simulink model "gm_uz_pmsm_model_nonlinear"  (R2023a)
settings: Solver=FixedStepAuto  StartTime=0.0  StopTime=0.5  RelTol=1e-3
PreLoadFcn:
  | uz_pmsm_model_init_parameter
PostLoadFcn:
  | % Import the data from Excel for a lookup table
  | FluxMapData = readtable('C:\Users\Philipp\ultrazohm\ultrazohm_sw\ip_cores\uz_pmsm_model\FluxMapData_2023-05-26_13-07-57.csv');
  | % Row indices for lookup table
  | d_current_in_d_axis = FluxMapData(8:27,1:end);
  | % Column indices for lookup table
  | q_current_in_d_axis = FluxMapData(29:48,1:end);
  | % Output values for lookup table
  | d_Flux_d_axis = FluxMapData(50:69,1:end);
undefined symbols (not defined in the file or in its folder): d_current_d_Flux, d_current_q_Flux, Flux_d, Flux_q, friction_coefficient, inertia, k_i_d, k_p_d, k_p_q, L_d, L_q, Ldd, Ldq, Lqd, Lqq, polepair, psi_pm, q_current_d_Flux, q_current_q_Flux, R_1, setpoint_step, simulate_mechanical, simulate_open_loop, static_friction_torque
libraries: hdlmdlgenlib x8, slpidlib x2
(part 1 of 2)
settings Model: Creator=ts  LastModifiedBy=Philipp
settings SolverCC: AlgebraicLoopSolver=TrustRegion  AutoInsertRateTranBlk=on
settings DataIOCC: LimitDataPoints=on  SaveOutput=off  SaveTime=off
settings OptimizationCC: BlockReduction=off  ConditionallyExecuteInputs=off  DefaultParameterBehavior=Inlined  LifeSpan=inf
settings DebuggingCC: AlgebraicLoopMsg=error  InheritedTsInSrcMsg=none  SingleTaskRateTransMsg=error  UnconnectedInputMsg=warning  UnconnectedOutputMsg=warning  UnconnectedLineMsg=warning  AllowSymbolicDim=off  StrictBusMsg=ErrorOnBusTreatedAsVector  SFUnexpectedBacktrackingDiag=warning  SFNoUnconditionalDefaultTransitionDiag=warning  SFExecutionAtInitializationDiag=none  ArithmeticOperatorsInVariantConditions=warning
settings HardwareCC: ProdBitPerPointer=32  ProdBitPerSizeT=32  ProdBitPerPtrDiffT=32  ProdLargestAtomicFloat=None  ProdIntDivRoundTo=Undefined  ProdEndianess=Unspecified  ProdWordSize=32  ProdHWDeviceType=ASIC/FPGA->ASIC/FPGA  ProdEqTarget=off
settings ModelReferenceCC: EnableRefExpFcnMdlSchedulingChecks=on
settings SFSimCC: SimUseLocalCustomCode=off  CustomCodeUndefinedFunction=UseInterfaceOnly
settings RTWCC: RTWUseLocalCustomCode=off  DLArmComputeVersion=19.05
settings CodeAppCC: StateflowObjectComments=on
settings GRTTargetCC: TargetLangStandard=C89/C90 (ANSI)
settings ConfigComp: CovScope=ReferencedModels  CovMetricSettings=dw  CovSaveCumulativeToWorkspaceVar=on  CovSaveSingleToWorkspaceVar=on  CovExternalEMLEnable=off  CovSFcnEnable=off

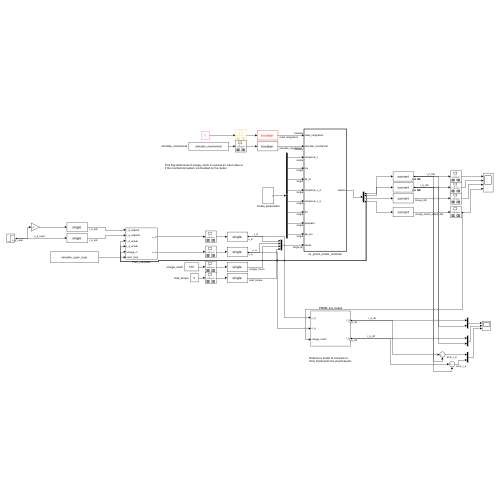
[thumbnail: Simulink's stored preview of the top-level diagram]
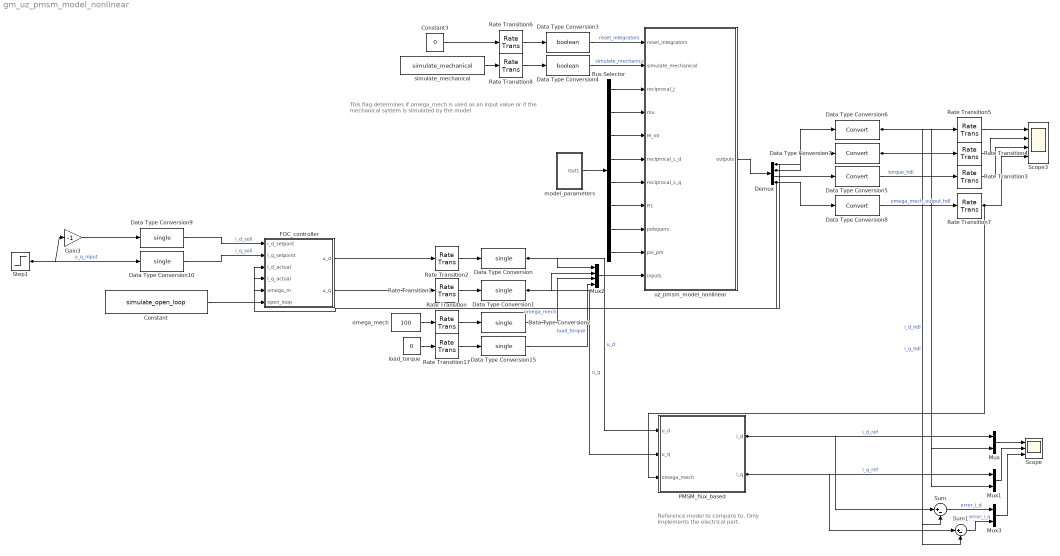
== system gm_uz_pmsm_model_nonlinear ==
  note: This flag determines if omega_mech is used as an input value or
      | if the mechanical system is simulated by the model
  note: Reference model to compare to.
      | Only implements the electrical part.
  Bus Selector : BusSelector  OutputSignals=1_J,mu,M_R0,1_L_d,1_L_q,R_1,polepair,psi_pm
  Constant : Constant  Value=simulate_open_loop
  Constant3 : Constant  Value=0
  Data Type Conversion{,1..2,9..10,15} (6 alike) : DataTypeConversion  OutDataTypeStr=single  SaturateOnIntegerOverflow=off  RndMeth=Floor
  Data Type Conversion3 : DataTypeConversion  OutDataTypeStr=boolean  SaturateOnIntegerOverflow=off  RndMeth=Floor
  Data Type Conversion4 : DataTypeConversion  OutDataTypeStr=boolean  SaturateOnIntegerOverflow=off  RndMeth=Floor
  Data Type Conversion{5..8} (4 alike) : DataTypeConversion  SaturateOnIntegerOverflow=off  RndMeth=Floor
  Demux : Demux
  FOC_controller : Subsystem
  Gain3 : Gain  Gain=-1
  Mux : Mux  Inputs=2
  Mux1 : Mux  Inputs=2
  Mux2 : Mux
  Mux3 : Mux  Inputs=2
  PMSM_flux_based : Subsystem
  Rate Transition{,1..2,6,8,17} (6 alike) : RateTransition  OutPortSampleTime=ts
  Rate Transition{3..5,7} (4 alike) : RateTransition
  Scope : Scope  NumInputPorts=3
  Scope3 : Scope  NumInputPorts=4
  Step1 : Step  Time=0.2  After=setpoint_step
  Sum : Sum  Inputs=|+-
  Sum1 : Sum  Inputs=|+-
  load_torque : Constant  Value=0
  model_parameters : Subsystem
  omega_mech : Constant  Value=100
  simulate_mechanical : Constant  Value=simulate_mechanical
  uz_pmsm_model_nonlinear : Subsystem  TreatAsAtomicUnit=on
  wires:
  Constant/1 -> FOC_controller/6(open_loop)
  omega_mech/1 -> Rate Transition/1
  FOC_controller/2(u_q) -> Rate Transition1/1
  FOC_controller/1(u_d) -> Rate Transition2/1
  Data Type Conversion10/1 -> FOC_controller/2(i_q_setpoint)  "i_q_soll"
  Data Type Conversion9/1 -> FOC_controller/1(i_d_setpont)  "i_d_soll"
  uz_pmsm_model_nonlinear/1(outputs) -> Demux/1
  Mux2/1 -> uz_pmsm_model_nonlinear/11(inputs)
  Data Type Conversion2/1 -> Mux2/3  "omega_mech"
  Data Type Conversion15/1 -> Mux2/4  "load_torque"
  Data Type Conversion1/1 -> Mux2/2, PMSM_flux_based/2(u_q)  "u_q"
  Data Type Conversion/1 -> Mux2/1, PMSM_flux_based/1(u_d)  "u_d"
  Demux/2 -> FOC_controller/4(i_q_actual), Data Type Conversion7/1
  Demux/4 -> FOC_controller/5(omega_m), Data Type Conversion8/1
  Demux/1 -> FOC_controller/3(i_d_actual), Data Type Conversion6/1
  Gain3/1 -> Data Type Conversion9/1
  Demux/3 -> Data Type Conversion5/1
  Step1/1 -> Data Type Conversion10/1, Gain3/1  "u_q_input"
  Mux3/1 -> Scope/3
  Sum1/1 -> Mux3/2  "error_i_q"
  Sum/1 -> Mux3/1  "error_i_d"
  model_parameters/1(Out1) -> Bus Selector/1
  Bus Selector/8 -> uz_pmsm_model_nonlinear/10(psi_pm)
  Bus Selector/7 -> uz_pmsm_model_nonlinear/9(polepairs)
  Bus Selector/6 -> uz_pmsm_model_nonlinear/8(R1)
  Bus Selector/5 -> uz_pmsm_model_nonlinear/7(reciprocal_L_q)
  Bus Selector/4 -> uz_pmsm_model_nonlinear/6(reciprocal_L_d)
  Bus Selector/3 -> uz_pmsm_model_nonlinear/5(M_n0)
  Bus Selector/2 -> uz_pmsm_model_nonlinear/4(mu)
  Bus Selector/1 -> uz_pmsm_model_nonlinear/3(reciprocal_J)
  Rate Transition7/1 -> Scope3/4, PMSM_flux_based/3(omega_mech)
  Data Type Conversion8/1 -> Rate Transition7/1  "omega_mech_output_hdl"
  PMSM_flux_based/1(i_d) -> Sum/1, Mux/1  "i_d_ref"
  PMSM_flux_based/2(i_q) -> Sum1/1, Mux1/1  "i_q_ref"
  Mux1/1 -> Scope/2
  Mux/1 -> Scope/1
  Rate Transition17/1 -> Data Type Conversion15/1
  load_torque/1 -> Rate Transition17/1
  Data Type Conversion4/1 -> uz_pmsm_model_nonlinear/2(simulate_mechanical)  "simulate_mechanics"
  Data Type Conversion3/1 -> uz_pmsm_model_nonlinear/1(reset_integrators)  "reset_integrators"
  simulate_mechanical/1 -> Rate Transition8/1
  Rate Transition8/1 -> Data Type Conversion4/1
  Constant3/1 -> Rate Transition6/1
  Rate Transition6/1 -> Data Type Conversion3/1
  Rate Transition3/1 -> Scope3/3
  Rate Transition5/1 -> Scope3/1
  Rate Transition4/1 -> Scope3/2
  Data Type Conversion5/1 -> Rate Transition3/1  "torque_hdl"
  Data Type Conversion7/1 -> Sum1/2, Mux1/2, Rate Transition4/1  "i_q_hdl"
  Data Type Conversion6/1 -> Rate Transition5/1, Sum/2, Mux/2  "i_d_hdl"
  Rate Transition2/1 -> Data Type Conversion/1
  Rate Transition1/1 -> Data Type Conversion1/1
  Rate Transition/1 -> Data Type Conversion2/1

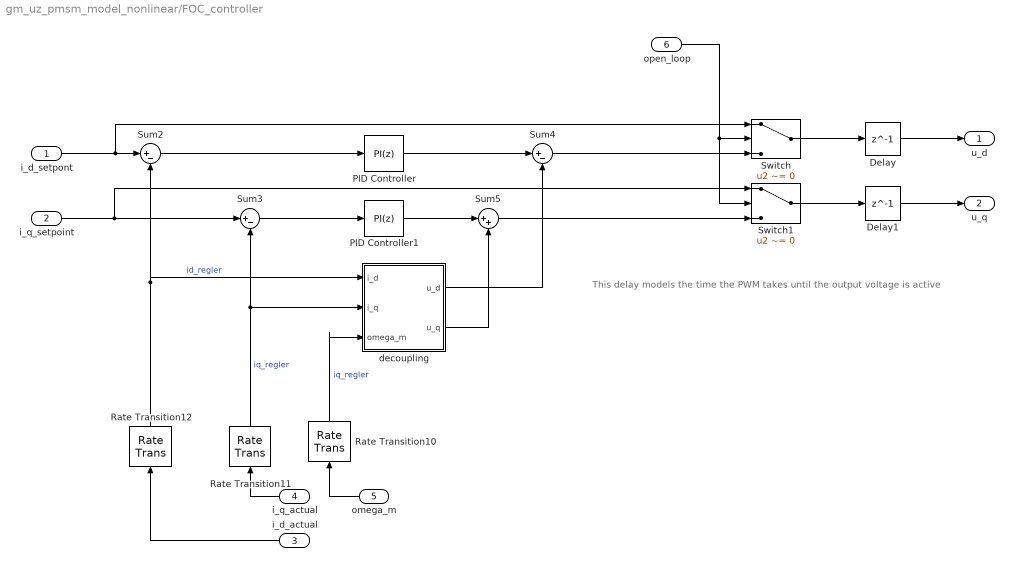
== system gm_uz_pmsm_model_nonlinear/FOC_controller ==
  note: This delay models the time the PWM takes until the output voltage is active
  i_d_setpont : Inport
  i_q_setpoint : Inport  Port=2
  i_d_actual : Inport  Port=3
  i_q_actual : Inport  Port=4
  omega_m : Inport  Port=5
  open_loop : Inport  Port=6
  Delay : Delay  DelayLength=1
  Delay1 : Delay  DelayLength=1
  PID Controller : slpidlib/PID Controller  Controller=PI  Form=Parallel  TimeDomain=Discrete-time  UseExternalTs=off  SampleTime=-1  IntegratorMethod=Forward Euler  FilterMethod=Forward Euler  ControllerParametersSource=internal  P=k_p_d  I=k_i_d  UseKiTs=off  D=0  N=100  UseFilter=on  TunerSelectOption=Transfer Function Based (PID Tuner App)  InitialConditionSource=internal  InitialConditionForIntegrator=0  InitialConditionForFilter=0  DifferentiatorICPrevScaledInput=0  ExternalReset=none  TrackingMode=off  Kt=1  LimitOutput=off  SatLimitsSource=internal  UpperSaturationLimit=inf  LowerSaturationLimit=-inf  LinearizeAsGain=on  AntiWindupMode=none  Kb=1  LimitIntegrator=off  UpperIntegratorSaturationLimit=inf  LowerIntegratorSaturationLimit=-inf  POutMin=[]  POutMax=[]  IOutMin=[]  IOutMax=[]  DOutMin=[]  DOutMax=[]  NOutMin=[]  NOutMax=[]  SumOutMin=[]  SumOutMax=[]  SaturationOutMin=[]  SaturationOutMax=[]  PParamMin=[]  PParamMax=[]  IParamMin=[]  IParamMax=[]  DParamMin=[]  DParamMax=[]  NParamMin=[]  NParamMax=[]  KbParamMin=[]  KbParamMax=[]  KtParamMin=[]  KtParamMax=[]  KbOutMin=[]  KbOutMax=[]  KtOutMin=[]  KtOutMax=[]  IntegratorOutMin=[]  IntegratorOutMax=[]  FilterOutMin=[]  FilterOutMax=[]  SumI1OutMin=[]  SumI1OutMax=[]  SumI2OutMin=[]  SumI2OutMax=[]  SumI3OutMin=[]  SumI3OutMax=[]  SumI4OutMin=[]  SumI4OutMax=[]  SumDOutMin=[]  SumDOutMax=[]  DifferentiatorOutMin=[]  DifferentiatorOutMax=[]  FilterDiffOutCoefMin=[]  FilterDiffOutCoefMax=[]  ReciprocalOutMin=[]  ReciprocalOutMax=[]  SumDenOutMin=[]  SumDenOutMax=[]  SumNumOutMin=[]  SumNumOutMax=[]  DivideOutMin=[]  DivideOutMax=[]  UdiffTsProdOutMin=[]  UdiffTsProdOutMax=[]  NTsProdOutMin=[]  NTsProdOutMax=[]  UintegralTsProdOutMin=[]  UintegralTsProdOutMax=[]  UngainTsProdOutMin=[]  UngainTsProdOutMax=[]  ClampingZeroOutDataTypeStr=Inherit: Inherit via back propagation  ClampingZeroOutMin=[]  ClampingZeroOutMax=[]  FilterDenConstantOutDataTypeStr=Inherit: Inherit via back propagation  FilterDenConstantOutMin=[]  FilterDenConstantOutMax=[]  PCopyOutDataTypeStr=Inherit: Inherit via back propagation  PCopyOutMin=[]  PCopyOutMax=[]  NCopyOutDataTypeStr=Inherit: Inherit via back propagation  NCopyOutMin=[]  NCopyOutMax=[]  IntegratorContinuousStateAttributes=''  IntegratorStateMustResolveToSignalObject=off  IntegratorRTWStateStorageClass=Auto  FilterContinuousStateAttributes=''  FilterStateMustResolveToSignalObject=off  FilterRTWStateStorageClass=Auto  ParallelPVariant=InternalParameters  IdealPVariant=Disabled  IVariant=InternalParameters  DVariant=Disabled  IntegratorVariant=Discrete  SatVariant=Disabled  AWVariant=Passthrough  PCopyVariant=Disabled  TRVariant=Disabled  FdbkBlocksVariant=Forward  IdealPFdbkVariant=Disabled  SatFdbkVariant=Disabled  DerivativeFilterVariant=Disabled  NVariant=Disabled  NCopyVariant=Disabled_SignalSpec  FilterICVariant=Disabled  IntegratorICVariant=InternalICs  ExternalResetVariant=Disabled  TRSumVariant=Passthrough  SumFdbkVariant=Disabled  SumVariant=Sum_PI  TsampFilterVariant=InternalTs  TsampNgainVariant=Passthrough  TsampIntegralVariant=Disabled_SignalSpec  ExternalSaturationOutDataTypeStr=Inherit: Same as second input
  PID Controller1 : slpidlib/PID Controller  Controller=PI  Form=Parallel  TimeDomain=Discrete-time  UseExternalTs=off  SampleTime=-1  IntegratorMethod=Forward Euler  FilterMethod=Forward Euler  ControllerParametersSource=internal  P=k_p_q  I=k_i_d  UseKiTs=off  D=0  N=100  UseFilter=on  TunerSelectOption=Transfer Function Based (PID Tuner App)  InitialConditionSource=internal  InitialConditionForIntegrator=0  InitialConditionForFilter=0  DifferentiatorICPrevScaledInput=0  ExternalReset=none  TrackingMode=off  Kt=1  LimitOutput=off  SatLimitsSource=internal  UpperSaturationLimit=inf  LowerSaturationLimit=-inf  LinearizeAsGain=on  AntiWindupMode=none  Kb=1  LimitIntegrator=off  UpperIntegratorSaturationLimit=inf  LowerIntegratorSaturationLimit=-inf  POutMin=[]  POutMax=[]  IOutMin=[]  IOutMax=[]  DOutMin=[]  DOutMax=[]  NOutMin=[]  NOutMax=[]  SumOutMin=[]  SumOutMax=[]  SaturationOutMin=[]  SaturationOutMax=[]  PParamMin=[]  PParamMax=[]  IParamMin=[]  IParamMax=[]  DParamMin=[]  DParamMax=[]  NParamMin=[]  NParamMax=[]  KbParamMin=[]  KbParamMax=[]  KtParamMin=[]  KtParamMax=[]  KbOutMin=[]  KbOutMax=[]  KtOutMin=[]  KtOutMax=[]  IntegratorOutMin=[]  IntegratorOutMax=[]  FilterOutMin=[]  FilterOutMax=[]  SumI1OutMin=[]  SumI1OutMax=[]  SumI2OutMin=[]  SumI2OutMax=[]  SumI3OutMin=[]  SumI3OutMax=[]  SumI4OutMin=[]  SumI4OutMax=[]  SumDOutMin=[]  SumDOutMax=[]  DifferentiatorOutMin=[]  DifferentiatorOutMax=[]  FilterDiffOutCoefMin=[]  FilterDiffOutCoefMax=[]  ReciprocalOutMin=[]  ReciprocalOutMax=[]  SumDenOutMin=[]  SumDenOutMax=[]  SumNumOutMin=[]  SumNumOutMax=[]  DivideOutMin=[]  DivideOutMax=[]  UdiffTsProdOutMin=[]  UdiffTsProdOutMax=[]  NTsProdOutMin=[]  NTsProdOutMax=[]  UintegralTsProdOutMin=[]  UintegralTsProdOutMax=[]  UngainTsProdOutMin=[]  UngainTsProdOutMax=[]  ClampingZeroOutDataTypeStr=Inherit: Inherit via back propagation  ClampingZeroOutMin=[]  ClampingZeroOutMax=[]  FilterDenConstantOutDataTypeStr=Inherit: Inherit via back propagation  FilterDenConstantOutMin=[]  FilterDenConstantOutMax=[]  PCopyOutDataTypeStr=Inherit: Inherit via back propagation  PCopyOutMin=[]  PCopyOutMax=[]  NCopyOutDataTypeStr=Inherit: Inherit via back propagation  NCopyOutMin=[]  NCopyOutMax=[]  IntegratorContinuousStateAttributes=''  IntegratorStateMustResolveToSignalObject=off  IntegratorRTWStateStorageClass=Auto  FilterContinuousStateAttributes=''  FilterStateMustResolveToSignalObject=off  FilterRTWStateStorageClass=Auto  ParallelPVariant=InternalParameters  IdealPVariant=Disabled  IVariant=InternalParameters  DVariant=Disabled  IntegratorVariant=Discrete  SatVariant=Disabled  AWVariant=Passthrough  PCopyVariant=Disabled  TRVariant=Disabled  FdbkBlocksVariant=Forward  IdealPFdbkVariant=Disabled  SatFdbkVariant=Disabled  DerivativeFilterVariant=Disabled  NVariant=Disabled  NCopyVariant=Disabled_SignalSpec  FilterICVariant=Disabled  IntegratorICVariant=InternalICs  ExternalResetVariant=Disabled  TRSumVariant=Passthrough  SumFdbkVariant=Disabled  SumVariant=Sum_PI  TsampFilterVariant=InternalTs  TsampNgainVariant=Passthrough  TsampIntegralVariant=Disabled_SignalSpec  ExternalSaturationOutDataTypeStr=Inherit: Same as second input
  Rate Transition10 : RateTransition  OutPortSampleTime=ts_regler
  Rate Transition11 : RateTransition  OutPortSampleTime=ts_regler
  Rate Transition12 : RateTransition  OutPortSampleTime=ts_regler
  Sum2 : Sum  Inputs=|+-
  Sum3 : Sum  Inputs=|+-
  Sum4 : Sum  Inputs=|+-
  Sum5 : Sum  Inputs=|++
  Switch : Switch  Criteria=u2 ~= 0  SaturateOnIntegerOverflow=off  InputSameDT=off
  Switch1 : Switch  Criteria=u2 ~= 0  SaturateOnIntegerOverflow=off  InputSameDT=off
  decoupling : Subsystem
  u_d : Outport
  u_q : Outport  Port=2
  wires:
  Delay1/1 -> u_q/1
  Delay/1 -> u_d/1
  Switch1/1 -> Delay1/1
  Switch/1 -> Delay/1
  decoupling/2(u_q) -> Sum5/2
  decoupling/1(u_d) -> Sum4/2
  Rate Transition10/1 -> decoupling/3(omega_m)  "iq_regler"
  open_loop/1 -> Switch/2, Switch1/2
  i_q_setpoint/1 -> Sum3/1, Switch1/1
  Rate Transition11/1 -> Sum3/2, decoupling/2(i_q)  "iq_regler"
  Rate Transition12/1 -> Sum2/2, decoupling/1(i_d)  "id_regler"
  i_q_actual/1 -> Rate Transition11/1
  Sum3/1 -> PID Controller1/1
  omega_m/1 -> Rate Transition10/1
  Sum5/1 -> Switch1/3
  Sum2/1 -> PID Controller/1
  i_d_setpont/1 -> Sum2/1, Switch/1
  i_d_actual/1 -> Rate Transition12/1
  Sum4/1 -> Switch/3
  PID Controller1/1 -> Sum5/1
  PID Controller/1 -> Sum4/1

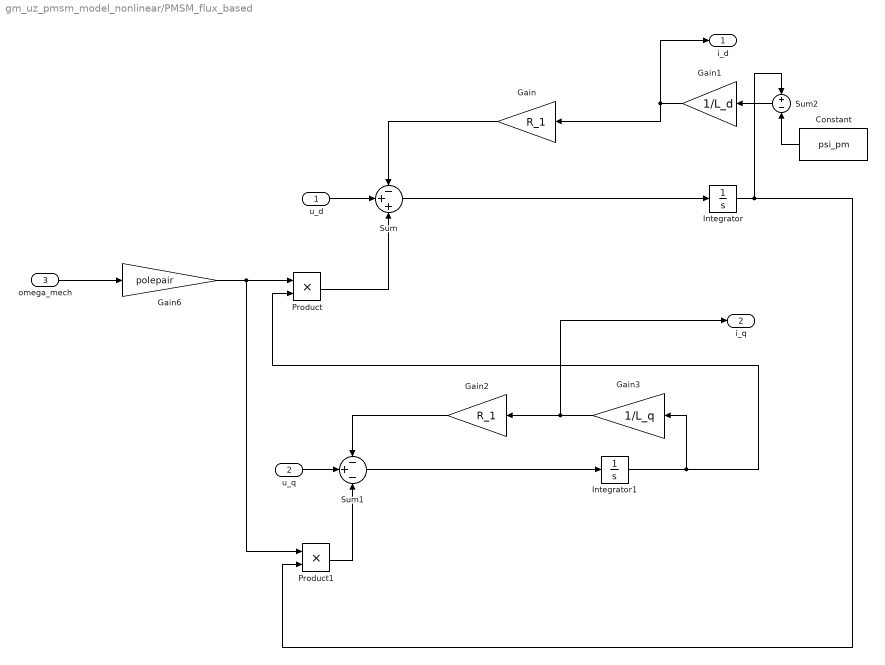
== system gm_uz_pmsm_model_nonlinear/PMSM_flux_based ==
  u_d : Inport
  u_q : Inport  Port=2
  omega_mech : Inport  Port=3
  Constant : Constant  Value=psi_pm
  Gain : Gain  Gain=R_1
  Gain1 : Gain  Gain=1/L_d
  Gain2 : Gain  Gain=R_1
  Gain3 : Gain  Gain=1/L_q
  Gain6 : Gain  Gain=polepair
  Integrator : Integrator
  Integrator1 : Integrator
  Product : Product
  Product1 : Product
  Sum : Sum  Inputs=-++
  Sum1 : Sum  Inputs=-+-
  Sum2 : Sum  Inputs=+-
  i_d : Outport
  i_q : Outport  Port=2
  wires:
  omega_mech/1 -> Gain6/1
  Gain3/1 -> Gain2/1, i_q/1
  Gain2/1 -> Sum1/1
  Sum1/1 -> Integrator1/1
  Product1/1 -> Sum1/3
  Integrator1/1 -> Product/2, Gain3/1
  Product/1 -> Sum/3
  Gain6/1 -> Product/1, Product1/1
  Gain1/1 -> i_d/1, Gain/1
  Sum2/1 -> Gain1/1
  Constant/1 -> Sum2/2
  Integrator/1 -> Sum2/1, Product1/2
  Gain/1 -> Sum/1
  Sum/1 -> Integrator/1
  u_q/1 -> Sum1/2
  u_d/1 -> Sum/2

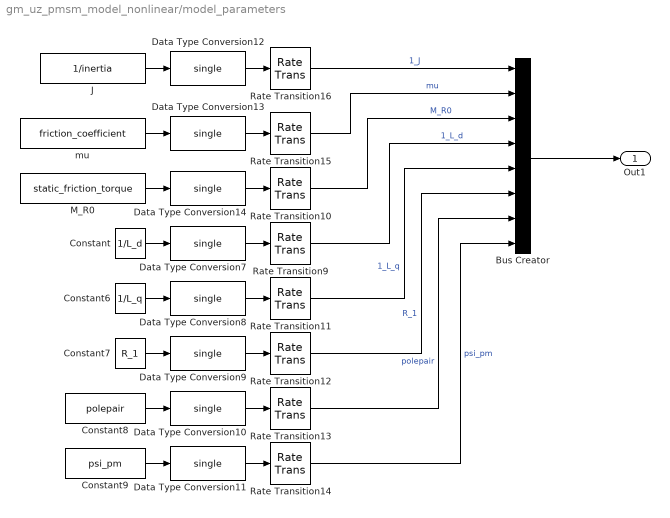
== system gm_uz_pmsm_model_nonlinear/model_parameters ==
  Bus Creator : BusCreator  Inputs=8
  Constant : Constant  Value=1/L_d
  Constant6 : Constant  Value=1/L_q
  Constant7 : Constant  Value=R_1
  Constant8 : Constant  Value=polepair
  Constant9 : Constant  Value=psi_pm
  Data Type Conversion{7..14} (8 alike) : DataTypeConversion  OutDataTypeStr=single  SaturateOnIntegerOverflow=off  RndMeth=Floor
  J : Constant  Value=1/inertia
  M_R0 : Constant  Value=static_friction_torque
  Rate Transition{9..16} (8 alike) : RateTransition  OutPortSampleTime=ts
  mu : Constant  Value=friction_coefficient
  Out1 : Outport
  wires:
  Constant/1 -> Data Type Conversion7/1
  Constant9/1 -> Data Type Conversion11/1
  Constant7/1 -> Data Type Conversion9/1
  Data Type Conversion13/1 -> Rate Transition15/1
  Rate Transition11/1 -> Bus Creator/5  "1_L_q"
  M_R0/1 -> Data Type Conversion14/1
  mu/1 -> Data Type Conversion13/1
  Data Type Conversion10/1 -> Rate Transition13/1
  Data Type Conversion8/1 -> Rate Transition11/1
  J/1 -> Data Type Conversion12/1
  Rate Transition9/1 -> Bus Creator/4  "1_L_d"
  Constant6/1 -> Data Type Conversion8/1
  Rate Transition15/1 -> Bus Creator/2  "mu"
  Data Type Conversion9/1 -> Rate Transition12/1
  Constant8/1 -> Data Type Conversion10/1
  Data Type Conversion11/1 -> Rate Transition14/1
  Bus Creator/1 -> Out1/1
  Rate Transition13/1 -> Bus Creator/7  "polepair"
  Rate Transition16/1 -> Bus Creator/1  "1_J"
  Rate Transition12/1 -> Bus Creator/6  "R_1"
  Data Type Conversion14/1 -> Rate Transition10/1
  Rate Transition14/1 -> Bus Creator/8  "psi_pm"
  Rate Transition10/1 -> Bus Creator/3  "M_R0"
  Data Type Conversion7/1 -> Rate Transition9/1
  Data Type Conversion12/1 -> Rate Transition16/1

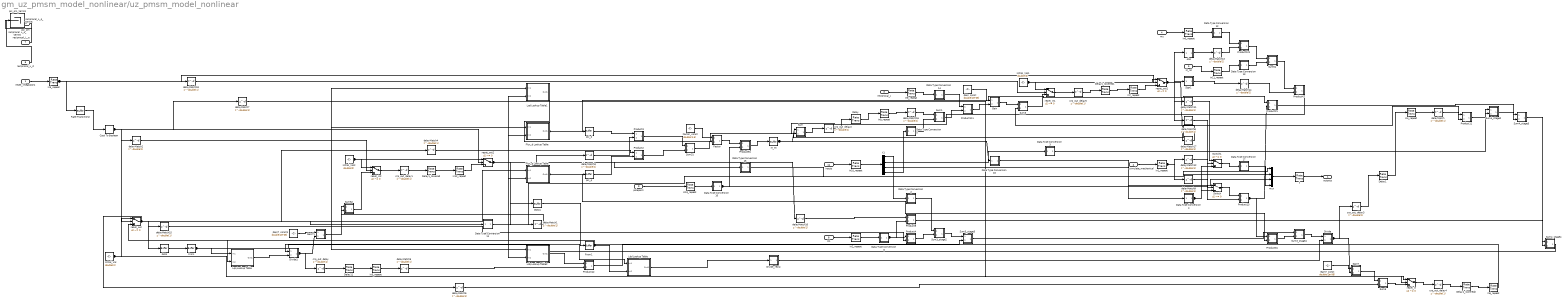
== system gm_uz_pmsm_model_nonlinear/uz_pmsm_model_nonlinear ==
  reset_integrators : Inport  OutDataTypeStr=boolean  PortDimensions=1  SampleTime=2e-06
  simulate_mechanical : Inport  Port=2  OutDataTypeStr=boolean  PortDimensions=1  SampleTime=2e-06
  reciprocal_J : Inport  Port=3  OutDataTypeStr=single  PortDimensions=1  SampleTime=2e-06
  mu : Inport  Port=4  OutDataTypeStr=single  PortDimensions=1  SampleTime=2e-06
  M_n0 : Inport  Port=5  OutDataTypeStr=single  PortDimensions=1  SampleTime=2e-06
  reciprocal_L_d : Inport  Port=6  OutDataTypeStr=single  PortDimensions=1  SampleTime=2e-06
  reciprocal_L_q : Inport  Port=7  OutDataTypeStr=single  PortDimensions=1  SampleTime=2e-06
  R1 : Inport  Port=8  OutDataTypeStr=single  PortDimensions=1  SampleTime=2e-06
  polepairs : Inport  Port=9  OutDataTypeStr=single  PortDimensions=1  SampleTime=2e-06
  psi_pm : Inport  Port=10  OutDataTypeStr=single  PortDimensions=1  SampleTime=2e-06
  inputs : Inport  Port=11  OutDataTypeStr=single  PortDimensions=[4]  SampleTime=2e-06
  Abs : Subsystem
      mask Display: disp('NFP\nabs');
  Cast To Boolean : DataTypeConversion  OutDataTypeStr=boolean
  Data Type Conversion10 : Subsystem
      mask Display: disp('NFP\nconv');
  Data Type Conversion11 : Subsystem
      mask Display: disp('NFP\nconv');
  Data Type Conversion12 : Subsystem
      mask Display: disp('NFP\nconv');
  Data Type Conversion13 : Subsystem
      mask Display: disp('NFP\nconv');
  Data Type Conversion14 : Subsystem
      mask Display: disp('NFP\nconv');
  Data Type Conversion15 : Subsystem
      mask Display: disp('NFP\nconv');
  Data Type Conversion16 : Subsystem
      mask Display: disp('NFP\nconv');
  Data Type Conversion17 : Subsystem
      mask Display: disp('NFP\nconv');
  Data Type Conversion2 : Subsystem
      mask Display: disp('NFP\nconv');
  Data Type Conversion3 : Subsystem
      mask Display: disp('NFP\nconv');
  Data Type Conversion4 : Subsystem
      mask Display: disp('NFP\nconv');
  Data Type Conversion5 : Subsystem
      mask Display: disp('NFP\nconv');
  Data Type Conversion6 : Subsystem
      mask Display: disp('NFP\nconv');
  Delay : RateTransition  OutPortSampleTimeOpt=Multiple of input port sample time  OutPortSampleTimeMultiple=200
  Delay1 : RateTransition  OutPortSampleTimeOpt=Multiple of input port sample time  OutPortSampleTimeMultiple=200
  Delay11 : RateTransition  OutPortSampleTimeOpt=Multiple of input port sample time  OutPortSampleTimeMultiple=200
  Delay1_lowered : RateTransition  OutPortSampleTimeOpt=Multiple of input port sample time  OutPortSampleTimeMultiple=200
  Delay1_lowered1 : RateTransition  OutPortSampleTimeOpt=Multiple of input port sample time  OutPortSampleTimeMultiple=200
  Delay1_lowered2 : RateTransition  OutPortSampleTimeOpt=Multiple of input port sample time  OutPortSampleTimeMultiple=200
  Divide : Subsystem
      mask Display: disp('NFP\nmul');
  Divide1 : Subsystem
      mask Display: disp('NFP\nmul');
  Divide_recip : Subsystem
      mask Display: disp('NFP\nmath');
  Factor : Subsystem
      mask Display: disp('NFP\nmul');
  Factor_const : Constant  Value=double(1.5)  OutDataTypeStr=double  SampleTime=1e-08
  Flux_d Lookup Table : Subsystem
  Flux_q Lookup Table : Subsystem
  From : hdlmdlgenlib/Buffer
  From1 : hdlmdlgenlib/Buffer
  Gain : Subsystem
      mask Display: disp('NFP\nmul');
  Gain7 : Subsystem
      mask Display: disp('NFP\nmul');
  Gain71 : Subsystem
      mask Display: disp('NFP\nmul');
  Gain7_const : Constant  Value=double(2e-06)  OutDataTypeStr=double  SampleTime=1e-08
  Gain7_const1 : Constant  Value=double(2e-06)  OutDataTypeStr=double  SampleTime=1e-08
  Gain_const : Constant  Value=double(2e-06)  OutDataTypeStr=double  SampleTime=1e-08
  Goto : hdlmdlgenlib/Buffer
  Goto1 : hdlmdlgenlib/Buffer
  Initial_Val : Constant  Value=double(0)  OutDataTypeStr=double  SampleTime=1e-08
  Initial_Val1 : Constant  Value=double(0)  OutDataTypeStr=double  SampleTime=1e-08
  Initial_Val2 : Constant  Value=double(0)  OutDataTypeStr=double  SampleTime=1e-08
  Ldd Lookup Table : Subsystem
  Ldq Lookup Table2 : Subsystem
  Lqd Lookup Table1 : Subsystem
  Lqq Lookup Table : Subsystem
  M_Mi : hdlmdlgenlib/Buffer
  Product11 : Subsystem
      mask Display: disp('NFP\nmul');
  Product111 : Subsystem
      mask Display: disp('NFP\nmul');
  Product12 : Subsystem
      mask Display: disp('NFP\nmul');
  Product121 : Subsystem
      mask Display: disp('NFP\nmul');
  Product13 : Subsystem
      mask Display: disp('NFP\nmul');
  Product2 : Subsystem
      mask Display: disp('NFP\nmul');
  Product21 : Subsystem
      mask Display: disp('NFP\nmul');
  Product3 : Subsystem
      mask Display: disp('NFP\nmul');
  Product31 : Subsystem
      mask Display: disp('NFP\nmul');
  Product4 : Subsystem
      mask Display: disp('NFP\nmul');
  Product41 : Subsystem
      mask Display: disp('NFP\nmul');
  Product9 : Subsystem
      mask Display: disp('NFP\nmul');
  Product91 : Subsystem
      mask Display: disp('NFP\nmul');
  Rate Transition2 : hdlmdlgenlib/Buffer
  Sign1 : Subsystem
      mask Display: disp('NFP\nsignum');
  Sum : Subsystem
      mask Display: disp('NFP\nadd');
  Sum1 : Subsystem
      mask Display: disp('NFP\nadd');
  Sum3 : Subsystem
      mask Display: disp('NFP\nadd');
  Sum31 : Subsystem
      mask Display: disp('NFP\nadd');
  Sum3_stage2 : Subsystem
      mask Display: disp('NFP\nadd');
  Sum3_stage3 : Subsystem
      mask Display: disp('NFP\nadd');
  Sum3_stage4 : Subsystem
      mask Display: disp('NFP\nadd');
  Sum4_stage2 : Subsystem
      mask Display: disp('NFP\nadd');
  Sum4_stage3 : Subsystem
      mask Display: disp('NFP\nadd');
  Sum4_stage4 : Subsystem
      mask Display: disp('NFP\nadd');
  Sum5 : Subsystem
      mask Display: disp('NFP\nadd');
  Sum51 : Subsystem
      mask Display: disp('NFP\nadd');
  Sum52 : Subsystem
      mask Display: disp('NFP\nadd');
  Switch : Switch  Criteria=u2 ~= 0  Threshold=double(0)  OutDataTypeStr=double  SampleTime=1e-08  SaturateOnIntegerOverflow=off  InputSameDT=off
  Switch1 : Switch  Criteria=u2 ~= 0  Threshold=double(0)  OutDataTypeStr=double  SampleTime=1e-08  SaturateOnIntegerOverflow=off  InputSameDT=off
  crp_out_delay{,1..5} (6 alike) : Delay  DelayLength=double(1)  InitialCondition=0  SampleTime=1e-08
  delayMatch{,1..18} (19 alike) : Delay  DelayLength=double(1)  InitialCondition=0  SampleTime=1e-08
  in0_repeat : RateTransition  Integrity=off  Deterministic=off  OutPortSampleTimeOpt=Multiple of input port sample time  OutPortSampleTimeMultiple=1/200
  in10_repeat : RateTransition  Integrity=off  Deterministic=off  OutPortSampleTimeOpt=Multiple of input port sample time  OutPortSampleTimeMultiple=1/200
  in11_repeat : RateTransition  Integrity=off  Deterministic=off  OutPortSampleTimeOpt=Multiple of input port sample time  OutPortSampleTimeMultiple=1/200
  in12_repeat : RateTransition  Integrity=off  Deterministic=off  OutPortSampleTimeOpt=Multiple of input port sample time  OutPortSampleTimeMultiple=1/200
  in13_repeat : RateTransition  Integrity=off  Deterministic=off  OutPortSampleTimeOpt=Multiple of input port sample time  OutPortSampleTimeMultiple=1/200
  in1_repeat : RateTransition  Integrity=off  Deterministic=off  OutPortSampleTimeOpt=Multiple of input port sample time  OutPortSampleTimeMultiple=1/200
  in2_repeat : RateTransition  Integrity=off  Deterministic=off  OutPortSampleTimeOpt=Multiple of input port sample time  OutPortSampleTimeMultiple=1/200
  in3_repeat : RateTransition  Integrity=off  Deterministic=off  OutPortSampleTimeOpt=Multiple of input port sample time  OutPortSampleTimeMultiple=1/200
  in4_repeat : RateTransition  Integrity=off  Deterministic=off  OutPortSampleTimeOpt=Multiple of input port sample time  OutPortSampleTimeMultiple=1/200
  in5_repeat : RateTransition  Integrity=off  Deterministic=off  OutPortSampleTimeOpt=Multiple of input port sample time  OutPortSampleTimeMultiple=1/200
  in6_repeat : RateTransition  Integrity=off  Deterministic=off  OutPortSampleTimeOpt=Multiple of input port sample time  OutPortSampleTimeMultiple=1/200
  in7_repeat : RateTransition  Integrity=off  Deterministic=off  OutPortSampleTimeOpt=Multiple of input port sample time  OutPortSampleTimeMultiple=1/200
  in8_repeat : RateTransition  Integrity=off  Deterministic=off  OutPortSampleTimeOpt=Multiple of input port sample time  OutPortSampleTimeMultiple=1/200
  in9_repeat : RateTransition  Integrity=off  Deterministic=off  OutPortSampleTimeOpt=Multiple of input port sample time  OutPortSampleTimeMultiple=1/200
  mux : Mux
  psi_d : hdlmdlgenlib/Buffer
  psi_pm_term9 : Terminator
  psi_q : hdlmdlgenlib/Buffer
  reciprocal_L_d_term5 : Terminator
  reciprocal_L_q_term6 : Terminator
  reset_in : Switch  Criteria=u2 ~= 0  Threshold=double(0)  OutDataTypeStr=double  SampleTime=1e-08  SaturateOnIntegerOverflow=off  InputSameDT=off
  reset_in1 : Switch  Criteria=u2 ~= 0  Threshold=double(0)  OutDataTypeStr=double  SampleTime=1e-08  SaturateOnIntegerOverflow=off  InputSameDT=off
  reset_in2 : Switch  Criteria=u2 ~= 0  Threshold=double(0)  OutDataTypeStr=double  SampleTime=1e-08  SaturateOnIntegerOverflow=off  InputSameDT=off
  reset_out : Switch  Criteria=u2 ~= 0  Threshold=double(0)  OutDataTypeStr=double  SampleTime=1e-08  SaturateOnIntegerOverflow=off  InputSameDT=off
  reset_out1 : Switch  Criteria=u2 ~= 0  Threshold=double(0)  OutDataTypeStr=double  SampleTime=1e-08  SaturateOnIntegerOverflow=off  InputSameDT=off
  reset_out2 : Switch  Criteria=u2 ~= 0  Threshold=double(0)  OutDataTypeStr=double  SampleTime=1e-08  SaturateOnIntegerOverflow=off  InputSameDT=off
  t : RateTransition  OutPortSampleTimeOpt=Multiple of input port sample time  OutPortSampleTimeMultiple=200
  t1 : Demux
  outputs : Outport  SampleTime=2e-06
  wires:
  reset_integrators/1 -> in5_repeat/1
  simulate_mechanical/1 -> in1_repeat/1
  reciprocal_J/1 -> in8_repeat/1
  mu/1 -> in0_repeat/1
  M_n0/1 -> in11_repeat/1
  reciprocal_L_d/1 -> reciprocal_L_d_term5/1
  reciprocal_L_q/1 -> reciprocal_L_q_term6/1
  R1/1 -> in2_repeat/1
  polepairs/1 -> in13_repeat/1
  psi_pm/1 -> psi_pm_term9/1
  inputs/1 -> in10_repeat/1
  t/1 -> outputs/1
  in0_repeat/1 -> Data Type Conversion12/1(In1)
  in1_repeat/1 -> delayMatch12/1, delayMatch9/1
  in2_repeat/1 -> Data Type Conversion6/1(In1)
  in5_repeat/1 -> delayMatch18/1, Rate Transition2/1, reset_out1/2
  in8_repeat/1 -> Data Type Conversion14/1(In1)
  in10_repeat/1 -> t1/1
  in11_repeat/1 -> Data Type Conversion13/1(In1)
  in13_repeat/1 -> Data Type Conversion10/1(In1)
  mux/1 -> t/1
  Delay1_lowered/1 -> in12_repeat/1
  in12_repeat/1 -> reset_out2/3
  Delay/1 -> in9_repeat/1
  in9_repeat/1 -> delayMatch16/1
  Delay1_lowered1/1 -> in7_repeat/1
  in7_repeat/1 -> reset_out1/3
  Delay1_lowered2/1 -> in6_repeat/1
  in6_repeat/1 -> reset_out/3
  Delay1/1 -> in4_repeat/1
  in4_repeat/1 -> delayMatch/1
  Delay11/1 -> in3_repeat/1
  in3_repeat/1 -> delayMatch5/1
  crp_out_delay/1 -> Delay11/1
  crp_out_delay1/1 -> Delay1_lowered/1
  crp_out_delay2/1 -> Delay/1
  crp_out_delay3/1 -> Delay1/1
  crp_out_delay4/1 -> Delay1_lowered2/1
  crp_out_delay5/1 -> Delay1_lowered1/1
  Data Type Conversion16/1(Out1) -> mux/3
  Data Type Conversion17/1(Out1) -> mux/4
  Switch1/1 -> Data Type Conversion17/1(In1)
  Lqq Lookup Table/1(Out1) -> Divide1/2(In2)
  Goto1/1 -> From1/1
  From1/1 -> Ldd Lookup Table/2(In2), Lqq Lookup Table/2(In2)
  Ldd Lookup Table/1(Out1) -> Divide_recip/1(In1)
  From/1 -> Ldd Lookup Table/1(In1), Lqq Lookup Table/1(In1)
  Goto/1 -> From/1
  psi_d/1 -> Product3/1(In1)
  Flux_d Lookup Table/1(Out1) -> Product21/1(In1), psi_d/1
  psi_q/1 -> Product2/2(In2)
  Product31/1(Out1) -> Sum3_stage4/2(In2)
  Flux_q Lookup Table/1(Out1) -> Product31/2(In2), psi_q/1
  Ldq Lookup Table2/1(Out1) -> Product12/1(In1)
  Lqd Lookup Table1/1(Out1) -> Product11/2(In2)
  delayMatch15/1 -> Product4/2(In2)
  Rate Transition2/1 -> Cast To Boolean/1
  Initial_Val/1 -> reset_out/1, reset_in/1
  reset_in/1 -> crp_out_delay4/1
  Divide/1(Out1) -> Gain7/2(In2), crp_out_delay3/1
  Data Type Conversion2/1(Out1) -> Sum3_stage2/1(In1)
  Data Type Conversion3/1(Out1) -> Sum4_stage2/1(In1)
  delayMatch17/1 -> Sum3/2(In2)
  Initial_Val1/1 -> reset_out1/1, reset_in1/1
  reset_in1/1 -> crp_out_delay5/1
  Data Type Conversion5/1(Out1) -> Sum1/2(In2)
  t1/1 -> Data Type Conversion2/1(In1)
  t1/2 -> Data Type Conversion3/1(In1)
  t1/3 -> Data Type Conversion4/1(In1)
  t1/4 -> Data Type Conversion5/1(In1)
  Data Type Conversion4/1(Out1) -> Switch/3, Switch1/3
  Switch/1 -> Product13/1(In1)
  delayMatch8/1 -> Switch/1
  delayMatch14/1 -> Product41/2(In2)
  delayMatch13/1 -> Product121/2(In2)
  M_Mi/1 -> Sum/1(In1), Data Type Conversion16/1(In1)
  Product91/1(Out1) -> M_Mi/1
  Factor/1(Out1) -> Product91/1(In1)
  delayMatch4/1 -> Product2/1(In1)
  Data Type Conversion15/1(Out1) -> mux/2
  delayMatch3/1 -> Product3/2(In2)
  delayMatch10/1 -> Product9/1(In1)
  Initial_Val2/1 -> reset_out2/1, reset_in2/1
  reset_in2/1 -> crp_out_delay1/1
  Divide1/1(Out1) -> Gain71/2(In2), crp_out_delay/1
  Product21/1(Out1) -> Sum4_stage3/2(In2)
  delayMatch5/1 -> Product12/2(In2)
  delayMatch/1 -> Product11/1(In1)
  Gain7_const/1 -> Gain7/1(In1)
  Gain_const/1 -> Gain/1(In1)
  Factor_const/1 -> Factor/1(In1)
  Gain7_const1/1 -> Gain71/1(In1)
  delayMatch9/1 -> Switch/2
  delayMatch18/1 -> reset_in1/2
  delayMatch16/1 -> Sum1/1(In1)
  reset_out2/1 -> delayMatch1/1, delayMatch10/1, Goto1/1, Flux_d Lookup Table/2(In2), Flux_q Lookup Table/2(In2), Ldq Lookup Table2/2(In2), Lqd Lookup Table1/2(In2), Data Type Conversion15/1(In1), delayMatch3/1
  reset_out/1 -> delayMatch6/1, delayMatch15/1, Goto/1, Flux_d Lookup Table/1(In1), Flux_q Lookup Table/1(In1), Ldq Lookup Table2/1(In1), Lqd Lookup Table1/1(In1), Data Type Conversion11/1(In1), delayMatch4/1
  Cast To Boolean/1 -> delayMatch7/1, delayMatch2/1, reset_out2/2, reset_out/2
  Data Type Conversion12/1(Out1) -> Product121/1(In1)
  Product9/1(Out1) -> Sum4_stage4/2(In2)
  Data Type Conversion6/1(Out1) -> Product4/1(In1), Product9/2(In2)
  Product4/1(Out1) -> Sum3_stage2/2(In2)
  Product3/1(Out1) -> Sum31/1(In1)
  Product12/1(Out1) -> Sum3_stage3/2(In2)
  Product11/1(Out1) -> Sum4_stage2/2(In2)
  Sum5/1(Out1) -> reset_in/3
  Divide_recip/1(Out1) -> Divide/2(In2)
  Sum3_stage2/1(Out1) -> Sum3_stage3/1(In1)
  Sum3_stage3/1(Out1) -> Sum3_stage4/1(In1)
  Sum3_stage4/1(Out1) -> Divide/1(In1)
  Sum3/1(Out1) -> reset_in1/3
  Data Type Conversion14/1(Out1) -> Product111/1(In1)
  Product111/1(Out1) -> Gain/2(In2)
  Sum1/1(Out1) -> Product111/2(In2)
  Sign1/1(Out1) -> delayMatch14/1
  Abs/1(Out1) -> delayMatch13/1
  Product121/1(Out1) -> Sum51/1(In1)
  Data Type Conversion13/1(Out1) -> Sum51/2(In2)
  Sum51/1(Out1) -> Product41/1(In1)
  Product41/1(Out1) -> Sum/2(In2)
  Sum/1(Out1) -> crp_out_delay2/1
  Sum31/1(Out1) -> Factor/2(In2)
  Product2/1(Out1) -> Sum31/2(In2)
  Data Type Conversion11/1(Out1) -> mux/1
  Sum52/1(Out1) -> reset_in2/3
  Sum4_stage2/1(Out1) -> Sum4_stage3/1(In1)
  Sum4_stage3/1(Out1) -> Sum4_stage4/1(In1)
  Sum4_stage4/1(Out1) -> Divide1/1(In1)
  Product13/1(Out1) -> Product21/2(In2), Product31/1(In1)
  Data Type Conversion10/1(Out1) -> Product13/2(In2), Product91/2(In2)
  Gain7/1(Out1) -> Sum5/1(In1)
  Gain/1(Out1) -> Sum3/1(In1)
  Gain71/1(Out1) -> Sum52/1(In1)
  delayMatch11/1 -> Switch1/1
  delayMatch12/1 -> Switch1/2
  delayMatch1/1 -> Sum52/2(In2)
  delayMatch2/1 -> reset_in2/2
  delayMatch6/1 -> Sum5/2(In2)
  delayMatch7/1 -> reset_in/2
  reset_out1/1 -> delayMatch17/1, Abs/1(In1), Sign1/1(In1), delayMatch11/1, delayMatch8/1

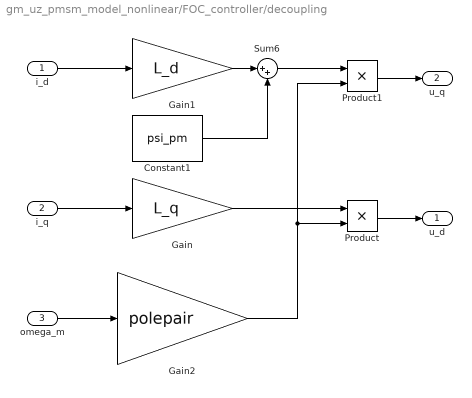
== system gm_uz_pmsm_model_nonlinear/FOC_controller/decoupling ==
  i_d : Inport
  i_q : Inport  Port=2
  omega_m : Inport  Port=3
  Constant1 : Constant  Value=psi_pm  SampleTime=-1
  Gain : Gain  Gain=L_q
  Gain1 : Gain  Gain=L_d
  Gain2 : Gain  Gain=polepair
  Product : Product
  Product1 : Product
  Sum6 : Sum  Inputs=|++
  u_d : Outport
  u_q : Outport  Port=2
  wires:
  omega_m/1 -> Gain2/1
  Sum6/1 -> Product1/1
  Constant1/1 -> Sum6/2
  i_q/1 -> Gain/1
  Gain1/1 -> Sum6/1
  Product/1 -> u_d/1
  i_d/1 -> Gain1/1
  Product1/1 -> u_q/1
  Gain2/1 -> Product/2, Product1/2
  Gain/1 -> Product/1

== system gm_uz_pmsm_model_nonlinear/uz_pmsm_model_nonlinear/Abs ==
  In1 : Inport
  Abs : Abs  SampleTime=1e-08  OutDataTypeStr=double  SaturateOnIntegerOverflow=off
  Out1 : Outport
  wires:
  In1/1 -> Abs/1
  Abs/1 -> Out1/1

== system gm_uz_pmsm_model_nonlinear/uz_pmsm_model_nonlinear/Data Type Conversion10 ==
  In1 : Inport
  Data Type Conversion10 : DataTypeConversion  OutDataTypeStr=double  RndMeth=Nearest  SampleTime=1e-08  SaturateOnIntegerOverflow=off
  Data Type Conversion10_pd1 : Delay  DelayLength=3
  Out1 : Outport
  wires:
  In1/1 -> Data Type Conversion10/1
  Data Type Conversion10/1 -> Data Type Conversion10_pd1/1
  Data Type Conversion10_pd1/1 -> Out1/1

== system gm_uz_pmsm_model_nonlinear/uz_pmsm_model_nonlinear/Data Type Conversion11 ==
  In1 : Inport
  Data Type Conversion11 : DataTypeConversion  OutDataTypeStr=single  RndMeth=Nearest  SampleTime=1e-08  SaturateOnIntegerOverflow=off
  Data Type Conversion11_pd1 : Delay  DelayLength=3
  Out1 : Outport
  wires:
  In1/1 -> Data Type Conversion11/1
  Data Type Conversion11/1 -> Data Type Conversion11_pd1/1
  Data Type Conversion11_pd1/1 -> Out1/1

== system gm_uz_pmsm_model_nonlinear/uz_pmsm_model_nonlinear/Data Type Conversion12 ==
  In1 : Inport
  Data Type Conversion12 : DataTypeConversion  OutDataTypeStr=double  RndMeth=Nearest  SampleTime=1e-08  SaturateOnIntegerOverflow=off
  Data Type Conversion12_pd1 : Delay  DelayLength=3
  Out1 : Outport
  wires:
  In1/1 -> Data Type Conversion12/1
  Data Type Conversion12/1 -> Data Type Conversion12_pd1/1
  Data Type Conversion12_pd1/1 -> Out1/1

== system gm_uz_pmsm_model_nonlinear/uz_pmsm_model_nonlinear/Data Type Conversion13 ==
  In1 : Inport
  Data Type Conversion13 : DataTypeConversion  OutDataTypeStr=double  RndMeth=Nearest  SampleTime=1e-08  SaturateOnIntegerOverflow=off
  Data Type Conversion13_pd1 : Delay  DelayLength=3
  Out1 : Outport
  wires:
  In1/1 -> Data Type Conversion13/1
  Data Type Conversion13/1 -> Data Type Conversion13_pd1/1
  Data Type Conversion13_pd1/1 -> Out1/1

== system gm_uz_pmsm_model_nonlinear/uz_pmsm_model_nonlinear/Data Type Conversion14 ==
  In1 : Inport
  Data Type Conversion14 : DataTypeConversion  OutDataTypeStr=double  RndMeth=Nearest  SampleTime=1e-08  SaturateOnIntegerOverflow=off
  Data Type Conversion14_pd1 : Delay  DelayLength=3
  Out1 : Outport
  wires:
  In1/1 -> Data Type Conversion14/1
  Data Type Conversion14/1 -> Data Type Conversion14_pd1/1
  Data Type Conversion14_pd1/1 -> Out1/1

== system gm_uz_pmsm_model_nonlinear/uz_pmsm_model_nonlinear/Data Type Conversion15 ==
  In1 : Inport
  Data Type Conversion15 : DataTypeConversion  OutDataTypeStr=single  RndMeth=Nearest  SampleTime=1e-08  SaturateOnIntegerOverflow=off
  Data Type Conversion15_pd1 : Delay  DelayLength=3
  Out1 : Outport
  wires:
  In1/1 -> Data Type Conversion15/1
  Data Type Conversion15/1 -> Data Type Conversion15_pd1/1
  Data Type Conversion15_pd1/1 -> Out1/1

== system gm_uz_pmsm_model_nonlinear/uz_pmsm_model_nonlinear/Data Type Conversion16 ==
  In1 : Inport
  Data Type Conversion16 : DataTypeConversion  OutDataTypeStr=single  RndMeth=Nearest  SampleTime=1e-08  SaturateOnIntegerOverflow=off
  Data Type Conversion16_pd1 : Delay  DelayLength=3
  Out1 : Outport
  wires:
  In1/1 -> Data Type Conversion16/1
  Data Type Conversion16/1 -> Data Type Conversion16_pd1/1
  Data Type Conversion16_pd1/1 -> Out1/1

== system gm_uz_pmsm_model_nonlinear/uz_pmsm_model_nonlinear/Data Type Conversion17 ==
  In1 : Inport
  Data Type Conversion17 : DataTypeConversion  OutDataTypeStr=single  RndMeth=Nearest  SampleTime=1e-08  SaturateOnIntegerOverflow=off
  Data Type Conversion17_pd1 : Delay  DelayLength=3
  Out1 : Outport
  wires:
  In1/1 -> Data Type Conversion17/1
  Data Type Conversion17/1 -> Data Type Conversion17_pd1/1
  Data Type Conversion17_pd1/1 -> Out1/1

== system gm_uz_pmsm_model_nonlinear/uz_pmsm_model_nonlinear/Data Type Conversion2 ==
  In1 : Inport
  Data Type Conversion2 : DataTypeConversion  OutDataTypeStr=double  RndMeth=Nearest  SampleTime=1e-08  SaturateOnIntegerOverflow=off
  Data Type Conversion2_pd1 : Delay  DelayLength=3
  Out1 : Outport
  wires:
  In1/1 -> Data Type Conversion2/1
  Data Type Conversion2/1 -> Data Type Conversion2_pd1/1
  Data Type Conversion2_pd1/1 -> Out1/1

== system gm_uz_pmsm_model_nonlinear/uz_pmsm_model_nonlinear/Data Type Conversion3 ==
  In1 : Inport
  Data Type Conversion3 : DataTypeConversion  OutDataTypeStr=double  RndMeth=Nearest  SampleTime=1e-08  SaturateOnIntegerOverflow=off
  Data Type Conversion3_pd1 : Delay  DelayLength=3
  Out1 : Outport
  wires:
  In1/1 -> Data Type Conversion3/1
  Data Type Conversion3/1 -> Data Type Conversion3_pd1/1
  Data Type Conversion3_pd1/1 -> Out1/1

== system gm_uz_pmsm_model_nonlinear/uz_pmsm_model_nonlinear/Data Type Conversion4 ==
  In1 : Inport
  Data Type Conversion4 : DataTypeConversion  OutDataTypeStr=double  RndMeth=Nearest  SampleTime=1e-08  SaturateOnIntegerOverflow=off
  Data Type Conversion4_pd1 : Delay  DelayLength=3
  Out1 : Outport
  wires:
  In1/1 -> Data Type Conversion4/1
  Data Type Conversion4/1 -> Data Type Conversion4_pd1/1
  Data Type Conversion4_pd1/1 -> Out1/1

== system gm_uz_pmsm_model_nonlinear/uz_pmsm_model_nonlinear/Data Type Conversion5 ==
  In1 : Inport
  Data Type Conversion5 : DataTypeConversion  OutDataTypeStr=double  RndMeth=Nearest  SampleTime=1e-08  SaturateOnIntegerOverflow=off
  Data Type Conversion5_pd1 : Delay  DelayLength=3
  Out1 : Outport
  wires:
  In1/1 -> Data Type Conversion5/1
  Data Type Conversion5/1 -> Data Type Conversion5_pd1/1
  Data Type Conversion5_pd1/1 -> Out1/1

== system gm_uz_pmsm_model_nonlinear/uz_pmsm_model_nonlinear/Data Type Conversion6 ==
  In1 : Inport
  Data Type Conversion6 : DataTypeConversion  OutDataTypeStr=double  RndMeth=Nearest  SampleTime=1e-08  SaturateOnIntegerOverflow=off
  Data Type Conversion6_pd1 : Delay  DelayLength=3
  Out1 : Outport
  wires:
  In1/1 -> Data Type Conversion6/1
  Data Type Conversion6/1 -> Data Type Conversion6_pd1/1
  Data Type Conversion6_pd1/1 -> Out1/1

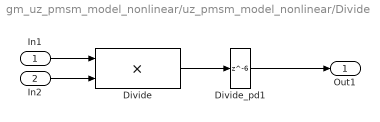
== system gm_uz_pmsm_model_nonlinear/uz_pmsm_model_nonlinear/Divide ==
  In1 : Inport
  In2 : Inport  Port=2
  Divide : Product  Inputs=**  OutDataTypeStr=double  SampleTime=1e-08
  Divide_pd1 : Delay  DelayLength=6
  Out1 : Outport
  wires:
  In1/1 -> Divide/1
  In2/1 -> Divide/2
  Divide/1 -> Divide_pd1/1
  Divide_pd1/1 -> Out1/1

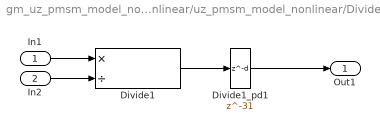
== system gm_uz_pmsm_model_nonlinear/uz_pmsm_model_nonlinear/Divide1 ==
  In1 : Inport
  In2 : Inport  Port=2
  Divide1 : Product  Inputs=*/  OutDataTypeStr=double  SampleTime=1e-08
  Divide1_pd1 : Delay  DelayLength=31
  Out1 : Outport
  wires:
  In1/1 -> Divide1/1
  In2/1 -> Divide1/2
  Divide1/1 -> Divide1_pd1/1
  Divide1_pd1/1 -> Out1/1

== system gm_uz_pmsm_model_nonlinear/uz_pmsm_model_nonlinear/Divide_recip ==
  In1 : Inport
  Divide_recip : Math  Operator=reciprocal  SampleTime=1e-08
  Divide_recip_pd1 : Delay  DelayLength=30
  Out1 : Outport
  wires:
  In1/1 -> Divide_recip/1
  Divide_recip/1 -> Divide_recip_pd1/1
  Divide_recip_pd1/1 -> Out1/1

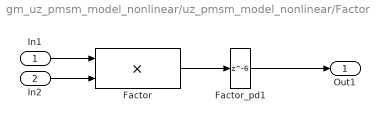
== system gm_uz_pmsm_model_nonlinear/uz_pmsm_model_nonlinear/Factor ==
  In1 : Inport
  In2 : Inport  Port=2
  Factor : Product  Inputs=**  OutDataTypeStr=double  SampleTime=1e-08
  Factor_pd1 : Delay  DelayLength=6
  Out1 : Outport
  wires:
  In1/1 -> Factor/1
  In2/1 -> Factor/2
  Factor/1 -> Factor_pd1/1
  Factor_pd1/1 -> Out1/1

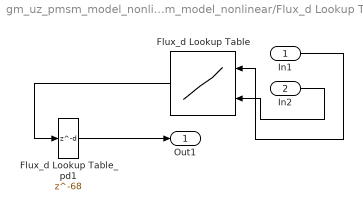
== system gm_uz_pmsm_model_nonlinear/uz_pmsm_model_nonlinear/Flux_d Lookup Table ==
  In1 : Inport
  In2 : Inport  Port=2
  Flux_d Lookup Table : Lookup_n-D  BreakpointsForDimension1=d_current_d_Flux  BreakpointsForDimension2=q_current_d_Flux  BreakpointsForDimension3=[5, 7]  Table=Flux_d  InternalRulePriority=Speed  RndMeth=Simplest
      settings: InputPortMap=u0,u1
  Flux_d Lookup Table_pd1 : Delay  DelayLength=68
  Out1 : Outport
  wires:
  Flux_d Lookup Table_pd1/1 -> Out1/1
  In2/1 -> Flux_d Lookup Table/2
  Flux_d Lookup Table/1 -> Flux_d Lookup Table_pd1/1
  In1/1 -> Flux_d Lookup Table/1

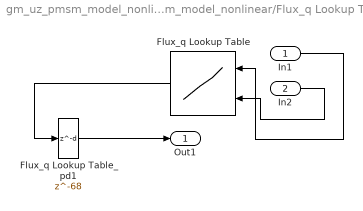
== system gm_uz_pmsm_model_nonlinear/uz_pmsm_model_nonlinear/Flux_q Lookup Table ==
  In1 : Inport
  In2 : Inport  Port=2
  Flux_q Lookup Table : Lookup_n-D  BreakpointsForDimension1=d_current_q_Flux  BreakpointsForDimension2=q_current_q_Flux  BreakpointsForDimension3=[5, 7]  Table=Flux_q  InternalRulePriority=Speed  RndMeth=Simplest
      settings: InputPortMap=u0,u1
  Flux_q Lookup Table_pd1 : Delay  DelayLength=68
  Out1 : Outport
  wires:
  In1/1 -> Flux_q Lookup Table/1
  Flux_q Lookup Table_pd1/1 -> Out1/1
  Flux_q Lookup Table/1 -> Flux_q Lookup Table_pd1/1
  In2/1 -> Flux_q Lookup Table/2

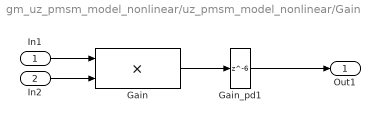
== system gm_uz_pmsm_model_nonlinear/uz_pmsm_model_nonlinear/Gain ==
  In1 : Inport
  In2 : Inport  Port=2
  Gain : Product  Inputs=**  OutDataTypeStr=double  SampleTime=1e-08
  Gain_pd1 : Delay  DelayLength=6
  Out1 : Outport
  wires:
  In1/1 -> Gain/1
  In2/1 -> Gain/2
  Gain/1 -> Gain_pd1/1
  Gain_pd1/1 -> Out1/1

== system gm_uz_pmsm_model_nonlinear/uz_pmsm_model_nonlinear/Gain7 ==
  In1 : Inport
  In2 : Inport  Port=2
  Gain7 : Product  Inputs=**  OutDataTypeStr=double  SampleTime=1e-08
  Gain7_pd1 : Delay  DelayLength=6
  Out1 : Outport
  wires:
  In1/1 -> Gain7/1
  In2/1 -> Gain7/2
  Gain7/1 -> Gain7_pd1/1
  Gain7_pd1/1 -> Out1/1

== system gm_uz_pmsm_model_nonlinear/uz_pmsm_model_nonlinear/Gain71 ==
  In1 : Inport
  In2 : Inport  Port=2
  Gain71 : Product  Inputs=**  OutDataTypeStr=double  SampleTime=1e-08
  Gain71_pd1 : Delay  DelayLength=6
  Out1 : Outport
  wires:
  In1/1 -> Gain71/1
  In2/1 -> Gain71/2
  Gain71/1 -> Gain71_pd1/1
  Gain71_pd1/1 -> Out1/1

== system gm_uz_pmsm_model_nonlinear/uz_pmsm_model_nonlinear/Ldd Lookup Table ==
  In1 : Inport
  In2 : Inport  Port=2
  Ldd Lookup Table : Lookup_n-D  BreakpointsForDimension1=d_current_q_Flux  BreakpointsForDimension2=q_current_q_Flux  BreakpointsForDimension3=[5, 7]  Table=Ldd  InternalRulePriority=Speed  RndMeth=Simplest
      settings: InputPortMap=u0,u1
  Ldd Lookup Table_pd1 : Delay  DelayLength=68
  Out1 : Outport
  wires:
  Ldd Lookup Table_pd1/1 -> Out1/1
  In1/1 -> Ldd Lookup Table/1
  In2/1 -> Ldd Lookup Table/2
  Ldd Lookup Table/1 -> Ldd Lookup Table_pd1/1

== system gm_uz_pmsm_model_nonlinear/uz_pmsm_model_nonlinear/Ldq Lookup Table2 ==
  In1 : Inport
  In2 : Inport  Port=2
  Ldq Lookup Table2 : Lookup_n-D  BreakpointsForDimension1=d_current_q_Flux  BreakpointsForDimension2=q_current_q_Flux  BreakpointsForDimension3=[5, 7]  Table=Ldq  InternalRulePriority=Speed  RndMeth=Simplest
      settings: InputPortMap=u0,u1
  Ldq Lookup Table2_pd1 : Delay  DelayLength=68
  Out1 : Outport
  wires:
  Ldq Lookup Table2_pd1/1 -> Out1/1
  Ldq Lookup Table2/1 -> Ldq Lookup Table2_pd1/1
  In1/1 -> Ldq Lookup Table2/1
  In2/1 -> Ldq Lookup Table2/2

== system gm_uz_pmsm_model_nonlinear/uz_pmsm_model_nonlinear/Lqd Lookup Table1 ==
  In1 : Inport
  In2 : Inport  Port=2
  Lqd Lookup Table1 : Lookup_n-D  BreakpointsForDimension1=d_current_q_Flux  BreakpointsForDimension2=q_current_q_Flux  BreakpointsForDimension3=[5, 7]  Table=Lqd  InternalRulePriority=Speed  RndMeth=Simplest
      settings: InputPortMap=u0,u1
  Lqd Lookup Table1_pd1 : Delay  DelayLength=68
  Out1 : Outport
  wires:
  Lqd Lookup Table1_pd1/1 -> Out1/1
  Lqd Lookup Table1/1 -> Lqd Lookup Table1_pd1/1
  In2/1 -> Lqd Lookup Table1/2
  In1/1 -> Lqd Lookup Table1/1

== system gm_uz_pmsm_model_nonlinear/uz_pmsm_model_nonlinear/Lqq Lookup Table ==
  In1 : Inport
  In2 : Inport  Port=2
  Lqq Lookup Table : Lookup_n-D  BreakpointsForDimension1=d_current_q_Flux  BreakpointsForDimension2=q_current_q_Flux  BreakpointsForDimension3=[5, 7]  Table=Lqq  InternalRulePriority=Speed  RndMeth=Simplest
      settings: InputPortMap=u0,u1
  Lqq Lookup Table_pd1 : Delay  DelayLength=68
  Out1 : Outport
  wires:
  In1/1 -> Lqq Lookup Table/1
  In2/1 -> Lqq Lookup Table/2
  Lqq Lookup Table/1 -> Lqq Lookup Table_pd1/1
  Lqq Lookup Table_pd1/1 -> Out1/1

== system gm_uz_pmsm_model_nonlinear/uz_pmsm_model_nonlinear/Product11 ==
  In1 : Inport
  In2 : Inport  Port=2
  Product11 : Product  Inputs=**  OutDataTypeStr=double  SampleTime=1e-08
  Product11_pd1 : Delay  DelayLength=6
  Out1 : Outport
  wires:
  In1/1 -> Product11/1
  In2/1 -> Product11/2
  Product11/1 -> Product11_pd1/1
  Product11_pd1/1 -> Out1/1

== system gm_uz_pmsm_model_nonlinear/uz_pmsm_model_nonlinear/Product111 ==
  In1 : Inport
  In2 : Inport  Port=2
  Product111 : Product  Inputs=**  OutDataTypeStr=double  SampleTime=1e-08
  Product111_pd1 : Delay  DelayLength=6
  Out1 : Outport
  wires:
  In1/1 -> Product111/1
  In2/1 -> Product111/2
  Product111/1 -> Product111_pd1/1
  Product111_pd1/1 -> Out1/1

== system gm_uz_pmsm_model_nonlinear/uz_pmsm_model_nonlinear/Product12 ==
  In1 : Inport
  In2 : Inport  Port=2
  Product12 : Product  Inputs=**  OutDataTypeStr=double  SampleTime=1e-08
  Product12_pd1 : Delay  DelayLength=6
  Out1 : Outport
  wires:
  In1/1 -> Product12/1
  In2/1 -> Product12/2
  Product12/1 -> Product12_pd1/1
  Product12_pd1/1 -> Out1/1

== system gm_uz_pmsm_model_nonlinear/uz_pmsm_model_nonlinear/Product121 ==
  In1 : Inport
  In2 : Inport  Port=2
  Product121 : Product  Inputs=**  OutDataTypeStr=double  SampleTime=1e-08
  Product121_pd1 : Delay  DelayLength=6
  Out1 : Outport
  wires:
  In1/1 -> Product121/1
  In2/1 -> Product121/2
  Product121/1 -> Product121_pd1/1
  Product121_pd1/1 -> Out1/1

== system gm_uz_pmsm_model_nonlinear/uz_pmsm_model_nonlinear/Product13 ==
  In1 : Inport
  In2 : Inport  Port=2
  Product13 : Product  Inputs=**  OutDataTypeStr=double  SampleTime=1e-08
  Product13_pd1 : Delay  DelayLength=6
  Out1 : Outport
  wires:
  In1/1 -> Product13/1
  In2/1 -> Product13/2
  Product13/1 -> Product13_pd1/1
  Product13_pd1/1 -> Out1/1

== system gm_uz_pmsm_model_nonlinear/uz_pmsm_model_nonlinear/Product2 ==
  In1 : Inport
  In2 : Inport  Port=2
  Product2 : Product  Inputs=**  OutDataTypeStr=double  SampleTime=1e-08
  Product2_pd1 : Delay  DelayLength=6
  Out1 : Outport
  wires:
  In1/1 -> Product2/1
  In2/1 -> Product2/2
  Product2/1 -> Product2_pd1/1
  Product2_pd1/1 -> Out1/1

== system gm_uz_pmsm_model_nonlinear/uz_pmsm_model_nonlinear/Product21 ==
  In1 : Inport
  In2 : Inport  Port=2
  Product21 : Product  Inputs=**  OutDataTypeStr=double  SampleTime=1e-08
  Product21_pd1 : Delay  DelayLength=6
  Out1 : Outport
  wires:
  In1/1 -> Product21/1
  In2/1 -> Product21/2
  Product21/1 -> Product21_pd1/1
  Product21_pd1/1 -> Out1/1

== system gm_uz_pmsm_model_nonlinear/uz_pmsm_model_nonlinear/Product3 ==
  In1 : Inport
  In2 : Inport  Port=2
  Product3 : Product  Inputs=**  OutDataTypeStr=double  SampleTime=1e-08
  Product3_pd1 : Delay  DelayLength=6
  Out1 : Outport
  wires:
  In1/1 -> Product3/1
  In2/1 -> Product3/2
  Product3/1 -> Product3_pd1/1
  Product3_pd1/1 -> Out1/1

== system gm_uz_pmsm_model_nonlinear/uz_pmsm_model_nonlinear/Product31 ==
  In1 : Inport
  In2 : Inport  Port=2
  Product31 : Product  Inputs=**  OutDataTypeStr=double  SampleTime=1e-08
  Product31_pd1 : Delay  DelayLength=6
  Out1 : Outport
  wires:
  In1/1 -> Product31/1
  In2/1 -> Product31/2
  Product31/1 -> Product31_pd1/1
  Product31_pd1/1 -> Out1/1

== system gm_uz_pmsm_model_nonlinear/uz_pmsm_model_nonlinear/Product4 ==
  In1 : Inport
  In2 : Inport  Port=2
  Product4 : Product  Inputs=**  OutDataTypeStr=double  SampleTime=1e-08
  Product4_pd1 : Delay  DelayLength=6
  Out1 : Outport
  wires:
  In1/1 -> Product4/1
  In2/1 -> Product4/2
  Product4/1 -> Product4_pd1/1
  Product4_pd1/1 -> Out1/1

== system gm_uz_pmsm_model_nonlinear/uz_pmsm_model_nonlinear/Product41 ==
  In1 : Inport
  In2 : Inport  Port=2
  Product41 : Product  Inputs=**  OutDataTypeStr=double  SampleTime=1e-08
  Product41_pd1 : Delay  DelayLength=6
  Out1 : Outport
  wires:
  In1/1 -> Product41/1
  In2/1 -> Product41/2
  Product41/1 -> Product41_pd1/1
  Product41_pd1/1 -> Out1/1

== system gm_uz_pmsm_model_nonlinear/uz_pmsm_model_nonlinear/Product9 ==
  In1 : Inport
  In2 : Inport  Port=2
  Product9 : Product  Inputs=**  OutDataTypeStr=double  SampleTime=1e-08
  Product9_pd1 : Delay  DelayLength=6
  Out1 : Outport
  wires:
  In1/1 -> Product9/1
  In2/1 -> Product9/2
  Product9/1 -> Product9_pd1/1
  Product9_pd1/1 -> Out1/1
